simulink model "MyVhclOperator_RTW"  (Simulink 7.5)
settings: Solver=ode1  SolverMode=SingleTasking  StartTime=0.0  StopTime=inf  FixedStep=0.001  RelTol=1e-3
PreLoadFcn:
  | vehicle = 'Car'; if ~length(which('cmcmd')), cmenv; end
  | MyVhclOperator_RTW_bus
InitFcn:
  | vehicle = 'Car'; if ~length(which('cmcmd')), cmenv; end
  | MyVhclOperator_RTW_bus
undefined symbols (not defined in the file or in its folder): OperationFinished, Phase, SteerAng, VCBus
libraries: simulink x45
(part 1 of 3)
Description:
  | CarMaker Real-Time Target (generic)
settings Model: Creator=ml  LastModifiedBy=ml
settings DebuggingCC: SolverPrmCheckMsg=none
settings HardwareCC: TargetHWDeviceType=32-bit Generic  ProdEqTarget=off
settings RTWCC: SystemTargetFile=CarMaker.tlc  TemplateMakefile=CarMaker_unix.tmf  Description=CarMaker Real-Time Target (32-bit)  ProcessScript=CarMaker_make_rtw_hook
settings CodeAppCC: MaxIdLength=127
settings STFCustomTargetCC: ModelReferenceCompliant=off  GeneratePreprocessorConditionals=Disable all  SystemTargetFile=CarMaker.tlc
settings GRTTargetCC: ModelReferenceCompliant=off  ParMdlRefBuildCompliant=off  CompOptLevelCompliant=off  MatFileLogging=off
settings CustomProperty: DataType=string  Value=..
settings EnumStrPairs: String=Car

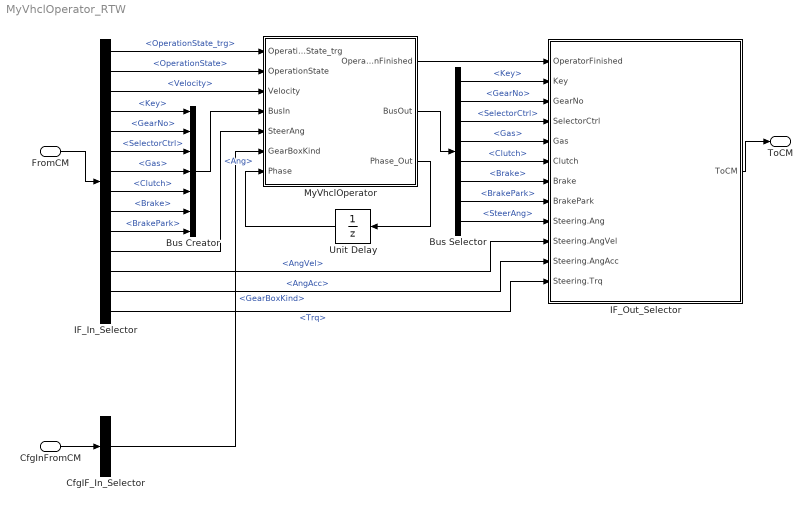
== system MyVhclOperator_RTW ==
  FromCM : Inport  UseBusObject=on
      settings: BusObject=cmVhclOperatorIn
  CfgInFromCM : Inport  Port=2  UseBusObject=on
      settings: BusObject=cmVhclOperatorCfgIn
  Bus Creator : BusCreator  Inputs=7
  Bus Selector : BusSelector  OutputSignals=VCBus.Key,VCBus.GearNo,VCBus.SelectorCtrl,VCBus.Gas,VCBus.Clutch,VCBus.Brake,VCBus.BrakePark,SteerAng
  CfgIF_In_Selector : BusSelector  OutputSignals=GearBoxKind
  IF_In_Selector : BusSelector  OutputSignals=OperationState_trg,OperationState,Velocity,Key,GearNo,SelectorCtrl,Gas,Clutch,Brake,BrakePark,Steering.Ang,Steering.AngVel,Steering.AngAcc,Steering.Trq
  IF_Out_Selector : Subsystem
      settings: OpenFcn=cmSignalSelect('SignalSelection_CB',gcb)
      mask Type: Signal Selection
      mask Description: Signal Selection Block
  MyVhclOperator : Subsystem
  Unit Delay : UnitDelay  SampleTime=-1
  ToCM : Outport  UseBusObject=on
      settings: BusObject=cmVhclOperatorOut
  wires:
  IF_In_Selector/1 -> MyVhclOperator/1(OperationState_trg)  "<OperationState_trg>"
  IF_Out_Selector/1(ToCM) -> ToCM/1
  CfgInFromCM/1 -> CfgIF_In_Selector/1
  CfgIF_In_Selector/1 -> MyVhclOperator/6(GearBoxKind)  "<GearBoxKind>"
  IF_In_Selector/2 -> MyVhclOperator/2(OperationState)  "<OperationState>"
  IF_In_Selector/3 -> MyVhclOperator/3(Velocity)  "<Velocity>"
  MyVhclOperator/3(Phase_Out) -> Unit Delay/1
  Unit Delay/1 -> MyVhclOperator/7(Phase)
  MyVhclOperator/1(OperationFinished) -> IF_Out_Selector/1(OperatorFinished)
  IF_In_Selector/4 -> Bus Creator/1  "<Key>"
  IF_In_Selector/5 -> Bus Creator/2  "<GearNo>"
  IF_In_Selector/6 -> Bus Creator/3  "<SelectorCtrl>"
  IF_In_Selector/7 -> Bus Creator/4  "<Gas>"
  IF_In_Selector/8 -> Bus Creator/5  "<Clutch>"
  IF_In_Selector/9 -> Bus Creator/6  "<Brake>"
  IF_In_Selector/10 -> Bus Creator/7  "<BrakePark>"
  IF_In_Selector/11 -> MyVhclOperator/5(SteerAng)  "<Ang>"
  FromCM/1 -> IF_In_Selector/1
  Bus Creator/1 -> MyVhclOperator/4(BusIn)
  MyVhclOperator/2(BusOut) -> Bus Selector/1
  Bus Selector/1 -> IF_Out_Selector/2(Key)  "<Key>"
  Bus Selector/2 -> IF_Out_Selector/3(GearNo)  "<GearNo>"
  Bus Selector/3 -> IF_Out_Selector/4(SelectorCtrl)  "<SelectorCtrl>"
  Bus Selector/4 -> IF_Out_Selector/5(Gas)  "<Gas>"
  Bus Selector/5 -> IF_Out_Selector/6(Clutch)  "<Clutch>"
  Bus Selector/6 -> IF_Out_Selector/7(Brake)  "<Brake>"
  Bus Selector/7 -> IF_Out_Selector/8(BrakePark)  "<BrakePark>"
  Bus Selector/8 -> IF_Out_Selector/9(Steering.Ang)  "<SteerAng>"
  IF_In_Selector/12 -> IF_Out_Selector/10(Steering.AngVel)  "<AngVel>"
  IF_In_Selector/13 -> IF_Out_Selector/11(Steering.AngAcc)  "<AngAcc>"
  IF_In_Selector/14 -> IF_Out_Selector/12(Steering.Trq)  "<Trq>"

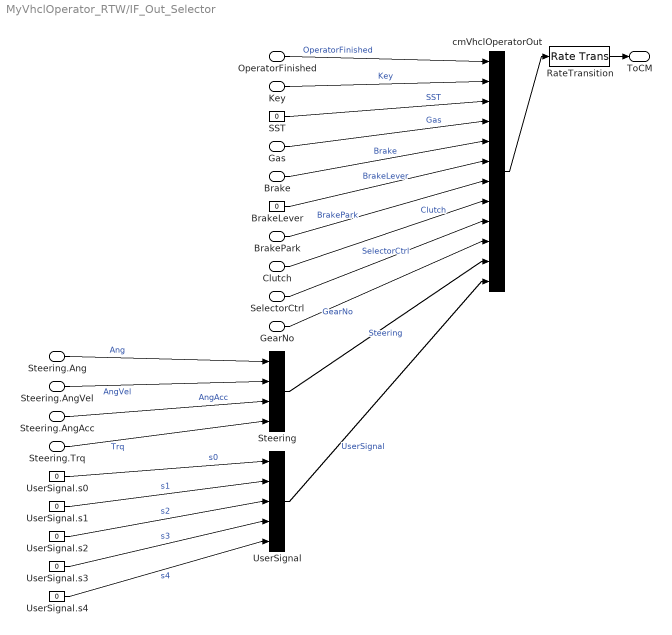
== system MyVhclOperator_RTW/IF_Out_Selector ==
  OperatorFinished : Inport
  Key : Inport  Port=2
  GearNo : Inport  Port=3
  SelectorCtrl : Inport  Port=4
  Gas : Inport  Port=5
  Clutch : Inport  Port=6
  Brake : Inport  Port=7
  BrakePark : Inport  Port=8
  Steering.Ang : Inport  Port=9
  Steering.AngVel : Inport  Port=10
  Steering.AngAcc : Inport  Port=11
  Steering.Trq : Inport  Port=12
  BrakeLever : Constant  Value=0
  RateTransition : RateTransition  OutPortSampleTime=str2num(get_param(bdroot,'FixedStep'))
  SST : Constant  Value=0
  Steering : BusCreator
  UserSignal : BusCreator  Inputs=5
  UserSignal.s{0..4} (5 alike) : Constant  Value=0
  cmVhclOperatorOut : BusCreator  Inputs=12
  ToCM : Outport
  wires:
  RateTransition/1 -> ToCM/1
  cmVhclOperatorOut/1 -> RateTransition/1
  SST/1 -> cmVhclOperatorOut/3  "SST"
  BrakeLever/1 -> cmVhclOperatorOut/6  "BrakeLever"
  Steering/1 -> cmVhclOperatorOut/11  "Steering"
  UserSignal/1 -> cmVhclOperatorOut/12  "UserSignal"
  UserSignal.s0/1 -> UserSignal/1  "s0"
  UserSignal.s1/1 -> UserSignal/2  "s1"
  UserSignal.s2/1 -> UserSignal/3  "s2"
  UserSignal.s3/1 -> UserSignal/4  "s3"
  UserSignal.s4/1 -> UserSignal/5  "s4"
  OperatorFinished/1 -> cmVhclOperatorOut/1  "OperatorFinished"
  Key/1 -> cmVhclOperatorOut/2  "Key"
  GearNo/1 -> cmVhclOperatorOut/10  "GearNo"
  SelectorCtrl/1 -> cmVhclOperatorOut/9  "SelectorCtrl"
  Gas/1 -> cmVhclOperatorOut/4  "Gas"
  Clutch/1 -> cmVhclOperatorOut/8  "Clutch"
  Brake/1 -> cmVhclOperatorOut/5  "Brake"
  BrakePark/1 -> cmVhclOperatorOut/7  "BrakePark"
  Steering.Ang/1 -> Steering/1  "Ang"
  Steering.AngVel/1 -> Steering/2  "AngVel"
  Steering.AngAcc/1 -> Steering/3  "AngAcc"
  Steering.Trq/1 -> Steering/4  "Trq"

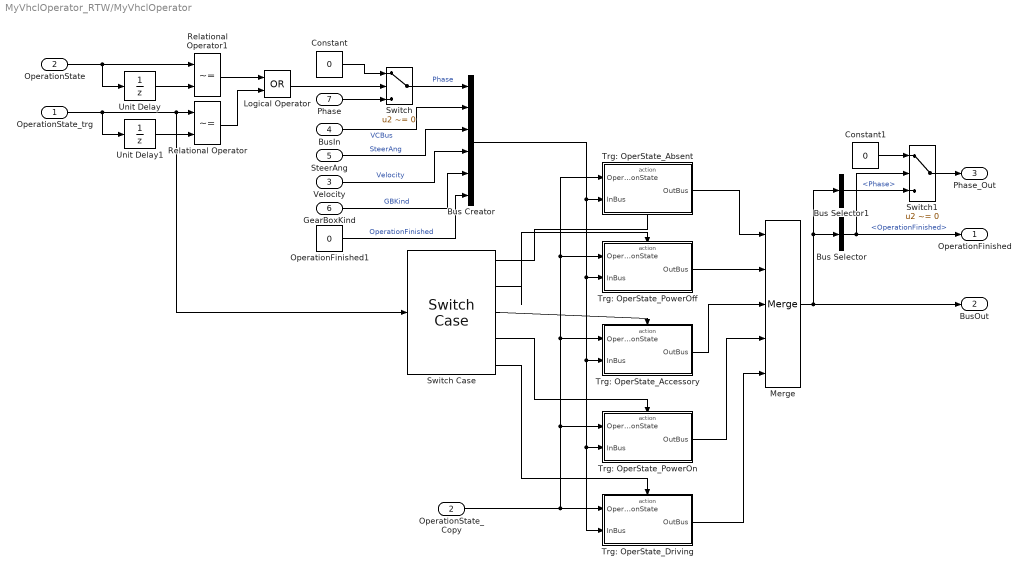
== system MyVhclOperator_RTW/MyVhclOperator ==
  OperationState_trg : Inport  OutDataType=fixdt(1, 16)  OutScaling=2^0
  OperationState : Inport  Port=2  OutDataType=fixdt(1, 16)  OutScaling=2^0
  Velocity : Inport  Port=3  OutDataType=fixdt(1, 16)  OutScaling=2^0
  BusIn : Inport  Port=4  OutDataType=fixdt(1, 16)  OutScaling=2^0
  SteerAng : Inport  Port=5  OutDataType=fixdt(1, 16)  OutScaling=2^0
  GearBoxKind : Inport  Port=6  OutDataType=fixdt(1, 16)  OutScaling=2^0
  Phase : Inport  Port=7  OutDataType=fixdt(1, 16)  OutScaling=2^0
  Bus Creator : BusCreator  Inputs=6
  Bus Selector : BusSelector  OutputSignals=OperationFinished
  Bus Selector1 : BusSelector  OutputSignals=Phase
  Constant : Constant  Value=0  OutDataType=fixdt(1, 16)  OutScaling=2^0
  Constant1 : Constant  Value=0  OutDataType=fixdt(1, 16)  OutScaling=2^0
  Logical Operator : Logic  Operator=OR  AllPortsSameDT=off  OutDataTypeMode=boolean  LogicDataType=fixdt(0, 8)  OutDataTypeStr=boolean
  Merge : Merge  Inputs=5
  OperationFinished1 : Constant  Value=0  OutDataType=fixdt(1, 16)  OutScaling=2^0
  OperationState_Copy : InportShadow  Port=2  OutDataType=fixdt(1, 16)  OutScaling=2^0
  Relational Operator : RelationalOperator  Operator=~=  LogicOutDataTypeMode=boolean  LogicDataType=fixdt(0, 8)  OutDataTypeStr=boolean
  Relational Operator1 : RelationalOperator  Operator=~=  LogicOutDataTypeMode=boolean  LogicDataType=fixdt(0, 8)  OutDataTypeStr=boolean
  Switch : Switch  Criteria=u2 ~= 0  OutDataType=fixdt(1, 16)  OutScaling=2^0
  Switch Case : SwitchCase  CaseConditions={0,1,2,3,4}  ShowDefaultCase=off
  Switch1 : Switch  Criteria=u2 ~= 0  OutDataType=fixdt(1, 16)  OutScaling=2^0
  Trg: OperState_Absent : Subsystem  TreatAsAtomicUnit=on
  Trg: OperState_Accessory : Subsystem  TreatAsAtomicUnit=on
  Trg: OperState_Driving : Subsystem  TreatAsAtomicUnit=on
  Trg: OperState_PowerOff : Subsystem  TreatAsAtomicUnit=on
  Trg: OperState_PowerOn : Subsystem  TreatAsAtomicUnit=on
  Unit Delay : UnitDelay  SampleTime=-1
  Unit Delay1 : UnitDelay  SampleTime=-1
  OperationFinished : Outport  OutDataType=fixdt(1, 16)  OutScaling=2^0
  BusOut : Outport  Port=2  OutDataType=fixdt(1, 16)  OutScaling=2^0
  Phase_Out : Outport  Port=3  OutDataType=fixdt(1, 16)  OutScaling=2^0
  wires:
  Switch/1 -> Bus Creator/1  "Phase"
  OperationState_trg/1 -> Relational Operator/1, Switch Case/1, Unit Delay1/1
  OperationState/1 -> Relational Operator1/1, Unit Delay/1
  Logical Operator/1 -> Switch/2
  Constant/1 -> Switch/1
  Switch Case/1 -> Trg: OperState_Absent/Action
  Switch Case/2 -> Trg: OperState_PowerOff/Action
  Switch Case/3 -> Trg: OperState_Accessory/Action
  Switch Case/4 -> Trg: OperState_PowerOn/Action
  Switch Case/5 -> Trg: OperState_Driving/Action
  Trg: OperState_Absent/1(OutBus) -> Merge/1
  Trg: OperState_PowerOff/1(OutBus) -> Merge/2
  Trg: OperState_Accessory/1(OutBus) -> Merge/3
  Trg: OperState_PowerOn/1(OutBus) -> Merge/4
  Trg: OperState_Driving/1(OutBus) -> Merge/5
  OperationState_Copy/1 -> Trg: OperState_PowerOff/1(OperationState), Trg: OperState_Absent/1(OperationState), Trg: OperState_Accessory/1(OperationState), Trg: OperState_PowerOn/1(OperationState), Trg: OperState_Driving/1(OperationState)
  Bus Creator/1 -> Trg: OperState_Absent/2(InBus), Trg: OperState_PowerOn/2(InBus), Trg: OperState_Driving/2(InBus), Trg: OperState_Accessory/2(InBus), Trg: OperState_PowerOff/2(InBus)
  Relational Operator1/1 -> Logical Operator/1
  Relational Operator/1 -> Logical Operator/2
  Unit Delay/1 -> Relational Operator1/2
  Unit Delay1/1 -> Relational Operator/2
  Phase/1 -> Switch/3
  BusIn/1 -> Bus Creator/2  "VCBus"
  SteerAng/1 -> Bus Creator/3  "SteerAng"
  Velocity/1 -> Bus Creator/4  "Velocity"
  GearBoxKind/1 -> Bus Creator/5  "GBKind"
  OperationFinished1/1 -> Bus Creator/6  "OperationFinished"
  Bus Selector/1 -> OperationFinished/1, Switch1/2  "<OperationFinished>"
  Switch1/1 -> Phase_Out/1
  Bus Selector1/1 -> Switch1/3  "<Phase>"
  Constant1/1 -> Switch1/1
  Merge/1 -> Bus Selector/1, Bus Selector1/1, BusOut/1

== system MyVhclOperator_RTW/MyVhclOperator/Trg: OperState_Absent ==
  note: Trg: OperState_Absent
  OperationState : Inport  OutDataType=fixdt(1, 16)  OutScaling=2^0
  InBus : Inport  Port=2  OutDataType=fixdt(1, 16)  OutScaling=2^0
  Action Port : ActionPort  ActionType=case
  Merge : Merge  Inputs=5
  OperState_Absent : Subsystem  TreatAsAtomicUnit=on
  OperState_Driving : Subsystem  TreatAsAtomicUnit=on
  OperState_PowerAccessory : Subsystem  TreatAsAtomicUnit=on
  OperState_PowerOff : Subsystem  TreatAsAtomicUnit=on
  OperState_PowerOn : Subsystem  TreatAsAtomicUnit=on
  Switch Case : SwitchCase  CaseConditions={0,1,2,3,4}  ShowDefaultCase=off
  OutBus : Outport  OutDataType=fixdt(1, 16)  OutScaling=2^0  InitialOutput=[0]
  wires:
  OperationState/1 -> Switch Case/1
  Switch Case/1 -> OperState_Absent/Action
  Switch Case/2 -> OperState_PowerOff/Action
  Switch Case/3 -> OperState_PowerAccessory/Action
  Switch Case/4 -> OperState_PowerOn/Action
  Switch Case/5 -> OperState_Driving/Action
  InBus/1 -> OperState_Absent/1(InBus), OperState_PowerOff/1(InBus), OperState_PowerAccessory/1(InBus), OperState_PowerOn/1(InBus), OperState_Driving/1(InBus)
  OperState_Absent/1(OutBus) -> Merge/1
  OperState_PowerOff/1(OutBus) -> Merge/2
  OperState_PowerAccessory/1(OutBus) -> Merge/3
  OperState_PowerOn/1(OutBus) -> Merge/4
  OperState_Driving/1(OutBus) -> Merge/5
  Merge/1 -> OutBus/1

== system MyVhclOperator_RTW/MyVhclOperator/Trg: OperState_Accessory ==
  note: Trg: OperState_Accessory
  OperationState : Inport  OutDataType=fixdt(1, 16)  OutScaling=2^0
  InBus : Inport  Port=2  OutDataType=fixdt(1, 16)  OutScaling=2^0
  Action Port : ActionPort  ActionType=case
  Merge : Merge  Inputs=5
  OperState_Absent : Subsystem  TreatAsAtomicUnit=on
  OperState_Accessory : Subsystem  TreatAsAtomicUnit=on
  OperState_Driving : Subsystem  TreatAsAtomicUnit=on
  OperState_PowerOff : Subsystem  TreatAsAtomicUnit=on
  OperState_PowerOn : Subsystem  TreatAsAtomicUnit=on
  Switch Case : SwitchCase  CaseConditions={0,1,2,3,4}  ShowDefaultCase=off
  OutBus : Outport  OutDataType=fixdt(1, 16)  OutScaling=2^0  InitialOutput=[0]
  wires:
  Merge/1 -> OutBus/1
  OperState_Driving/1(OutBus) -> Merge/5
  OperState_PowerOn/1(OutBus) -> Merge/4
  OperState_Accessory/1(OutBus) -> Merge/3
  OperState_PowerOff/1(OutBus) -> Merge/2
  OperState_Absent/1(OutBus) -> Merge/1
  InBus/1 -> OperState_PowerOff/1(InBus), OperState_Absent/1(InBus), OperState_Accessory/1(InBus), OperState_PowerOn/1(InBus), OperState_Driving/1(InBus)
  Switch Case/5 -> OperState_Driving/Action
  Switch Case/4 -> OperState_PowerOn/Action
  Switch Case/3 -> OperState_Accessory/Action
  Switch Case/2 -> OperState_PowerOff/Action
  Switch Case/1 -> OperState_Absent/Action
  OperationState/1 -> Switch Case/1

== system MyVhclOperator_RTW/MyVhclOperator/Trg: OperState_Driving ==
  note: Trg: OperState_Driving
  OperationState : Inport  OutDataType=fixdt(1, 16)  OutScaling=2^0
  InBus : Inport  Port=2  OutDataType=fixdt(1, 16)  OutScaling=2^0
  Action Port : ActionPort  ActionType=case
  Merge : Merge  Inputs=5
  OperState_Absent : Subsystem  TreatAsAtomicUnit=on
  OperState_Driving : Subsystem  TreatAsAtomicUnit=on
  OperState_PowerAccessory : Subsystem  TreatAsAtomicUnit=on
  OperState_PowerOff : Subsystem  TreatAsAtomicUnit=on
  OperState_PowerOn : Subsystem  TreatAsAtomicUnit=on
  Switch Case : SwitchCase  CaseConditions={0,1,2,3,4}  ShowDefaultCase=off
  OutBus : Outport  OutDataType=fixdt(1, 16)  OutScaling=2^0  InitialOutput=[0]
  wires:
  Merge/1 -> OutBus/1
  OperState_Driving/1(OutBus) -> Merge/5
  OperState_PowerOn/1(OutBus) -> Merge/4
  OperState_PowerAccessory/1(OutBus) -> Merge/3
  OperState_PowerOff/1(OutBus) -> Merge/2
  OperState_Absent/1(OutBus) -> Merge/1
  InBus/1 -> OperState_Absent/1(InBus), OperState_PowerOff/1(InBus), OperState_PowerAccessory/1(InBus), OperState_PowerOn/1(InBus), OperState_Driving/1(InBus)
  Switch Case/5 -> OperState_Driving/Action
  Switch Case/4 -> OperState_PowerOn/Action
  Switch Case/3 -> OperState_PowerAccessory/Action
  Switch Case/2 -> OperState_PowerOff/Action
  Switch Case/1 -> OperState_Absent/Action
  OperationState/1 -> Switch Case/1

== system MyVhclOperator_RTW/MyVhclOperator/Trg: OperState_PowerOff ==
  note: Trg: OperState_PowerOff
  OperationState : Inport  OutDataType=fixdt(1, 16)  OutScaling=2^0
  InBus : Inport  Port=2  OutDataType=fixdt(1, 16)  OutScaling=2^0
  Action Port : ActionPort  ActionType=case
  Merge : Merge  Inputs=5
  OperState_Absent : Subsystem  TreatAsAtomicUnit=on
  OperState_Driving : Subsystem  TreatAsAtomicUnit=on
  OperState_PowerAccessory : Subsystem  TreatAsAtomicUnit=on
  OperState_PowerOff : Subsystem  TreatAsAtomicUnit=on
  OperState_PowerOn : Subsystem  TreatAsAtomicUnit=on
  Switch Case : SwitchCase  CaseConditions={0,1,2,3,4}  ShowDefaultCase=off
  OutBus : Outport  OutDataType=fixdt(1, 16)  OutScaling=2^0  InitialOutput=[0]
  wires:
  OperationState/1 -> Switch Case/1
  Switch Case/1 -> OperState_Absent/Action
  Switch Case/2 -> OperState_PowerOff/Action
  Switch Case/3 -> OperState_PowerAccessory/Action
  Switch Case/4 -> OperState_PowerOn/Action
  Switch Case/5 -> OperState_Driving/Action
  InBus/1 -> OperState_PowerOff/1(InBus), OperState_Absent/1(InBus), OperState_PowerAccessory/1(InBus), OperState_PowerOn/1(InBus), OperState_Driving/1(InBus)
  OperState_Absent/1(OutBus) -> Merge/1
  OperState_PowerOff/1(OutBus) -> Merge/2
  OperState_PowerAccessory/1(OutBus) -> Merge/3
  OperState_PowerOn/1(OutBus) -> Merge/4
  OperState_Driving/1(OutBus) -> Merge/5
  Merge/1 -> OutBus/1

== system MyVhclOperator_RTW/MyVhclOperator/Trg: OperState_PowerOn ==
  note: Trg: OperState_PowerOn
  OperationState : Inport  OutDataType=fixdt(1, 16)  OutScaling=2^0
  InBus : Inport  Port=2  OutDataType=fixdt(1, 16)  OutScaling=2^0
  Action Port : ActionPort  ActionType=case
  Merge : Merge  Inputs=5
  OperState_Absent : Subsystem  TreatAsAtomicUnit=on
  OperState_Driving : Subsystem  TreatAsAtomicUnit=on
  OperState_PowerAccessory : Subsystem  TreatAsAtomicUnit=on
  OperState_PowerOff : Subsystem  TreatAsAtomicUnit=on
  OperState_PowerOn : Subsystem  TreatAsAtomicUnit=on
  Switch Case : SwitchCase  CaseConditions={0,1,2,3,4}  ShowDefaultCase=off
  OutBus : Outport  OutDataType=fixdt(1, 16)  OutScaling=2^0  InitialOutput=[0]
  wires:
  OperationState/1 -> Switch Case/1
  Switch Case/1 -> OperState_Absent/Action
  Switch Case/2 -> OperState_PowerOff/Action
  Switch Case/3 -> OperState_PowerAccessory/Action
  Switch Case/4 -> OperState_PowerOn/Action
  Switch Case/5 -> OperState_Driving/Action
  InBus/1 -> OperState_PowerOn/1(InBus), OperState_PowerAccessory/1(InBus), OperState_Absent/1(InBus), OperState_PowerOff/1(InBus), OperState_Driving/1(InBus)
  OperState_Absent/1(OutBus) -> Merge/1
  OperState_PowerOff/1(OutBus) -> Merge/2
  OperState_PowerAccessory/1(OutBus) -> Merge/3
  OperState_PowerOn/1(OutBus) -> Merge/4
  OperState_Driving/1(OutBus) -> Merge/5
  Merge/1 -> OutBus/1

== system MyVhclOperator_RTW/MyVhclOperator/Trg: OperState_Absent/OperState_Absent ==
  InBus : Inport  OutDataType=fixdt(1, 16)  OutScaling=2^0
  Action Port : ActionPort  ActionType=case
  Bus Assignment : BusAssignment  AssignedSignals=VCBus.Key,VCBus.GearNo,VCBus.SelectorCtrl,VCBus.Gas,VCBus.Clutch,VCBus.Brake,VCBus.BrakePark,Phase,OperationFinished
  Bus Selector : BusSelector  OutputSignals=GBKind
  Bus Selector1 : BusSelector  OutputSignals=Key,GearNo,SelectorCtrl,Gas,Clutch,Brake,BrakePark
  OperState: Absent : Subsystem
  OperationFinished : Constant  OutDataType=fixdt(1, 16)  OutScaling=2^0
  Phase : Constant  Value=0  OutDataType=fixdt(1, 16)  OutScaling=2^0
  Signal Conversion : SignalConversion  ConversionOutput=Bus copy
  OutBus : Outport  OutDataType=fixdt(1, 16)  OutScaling=2^0  InitialOutput=[0]
  wires:
  InBus/1 -> Bus Selector/1, Signal Conversion/1
  Bus Selector/1 -> OperState: Absent/1(GBKind)  "<GBKind>"
  Bus Assignment/1 -> OutBus/1
  OperationFinished/1 -> Bus Assignment/10
  Phase/1 -> Bus Assignment/9
  OperState: Absent/1(BusOut) -> Bus Selector1/1  "VC_Bus"
  Signal Conversion/1 -> Bus Assignment/1
  Bus Selector1/1 -> Bus Assignment/2  "<Key>"
  Bus Selector1/2 -> Bus Assignment/3  "<GearNo>"
  Bus Selector1/3 -> Bus Assignment/4  "<SelectorCtrl>"
  Bus Selector1/4 -> Bus Assignment/5  "<Gas>"
  Bus Selector1/5 -> Bus Assignment/6  "<Clutch>"
  Bus Selector1/6 -> Bus Assignment/7  "<Brake>"
  Bus Selector1/7 -> Bus Assignment/8  "<BrakePark>"

== system MyVhclOperator_RTW/MyVhclOperator/Trg: OperState_Absent/OperState_Driving ==
  InBus : Inport  OutDataType=fixdt(1, 16)  OutScaling=2^0
  Action Port : ActionPort  ActionType=case
  Drive2Off : Subsystem
  OutBus : Outport  OutDataType=fixdt(1, 16)  OutScaling=2^0
  wires:
  Drive2Off/1(BusOut) -> OutBus/1
  InBus/1 -> Drive2Off/1(BusIn)

== system MyVhclOperator_RTW/MyVhclOperator/Trg: OperState_Absent/OperState_PowerAccessory ==
  InBus : Inport  OutDataType=fixdt(1, 16)  OutScaling=2^0
  Action Port : ActionPort  ActionType=case
  Bus Assignment1 : BusAssignment  AssignedSignals=VCBus.Key,VCBus.GearNo,VCBus.SelectorCtrl,VCBus.Gas,VCBus.Clutch,VCBus.Brake,VCBus.BrakePark,Phase
  Bus Selector : BusSelector  OutputSignals=GBKind,Phase
  Bus Selector1 : BusSelector  OutputSignals=Key,GearNo,SelectorCtrl,Gas,Clutch,Brake,BrakePark
  OperState: PowerOn : Subsystem
  SetOutputAndWait : Subsystem
  Signal Conversion : SignalConversion  ConversionOutput=Bus copy
  OutBus : Outport  OutDataType=fixdt(1, 16)  OutScaling=2^0  InitialOutput=[0]
  wires:
  InBus/1 -> Bus Selector/1, Signal Conversion/1
  Bus Selector/1 -> OperState: PowerOn/1(GBKind)  "<GBKind>"
  Bus Assignment1/1 -> OutBus/1
  Bus Selector/2 -> SetOutputAndWait/1(PhaseIn)  "<Phase>"
  OperState: PowerOn/1(BusOut) -> Bus Selector1/1  "VC_Bus"
  SetOutputAndWait/1(PhaseOut) -> Bus Assignment1/9
  Signal Conversion/1 -> Bus Assignment1/1
  Bus Selector1/1 -> Bus Assignment1/2  "<Key>"
  Bus Selector1/2 -> Bus Assignment1/3  "<GearNo>"
  Bus Selector1/3 -> Bus Assignment1/4  "<SelectorCtrl>"
  Bus Selector1/4 -> Bus Assignment1/5  "<Gas>"
  Bus Selector1/5 -> Bus Assignment1/6  "<Clutch>"
  Bus Selector1/6 -> Bus Assignment1/7  "<Brake>"
  Bus Selector1/7 -> Bus Assignment1/8  "<BrakePark>"

== system MyVhclOperator_RTW/MyVhclOperator/Trg: OperState_Absent/OperState_PowerOff ==
  InBus : Inport  OutDataType=fixdt(1, 16)  OutScaling=2^0
  Action Port : ActionPort  ActionType=case
  Bus Assignment1 : BusAssignment  AssignedSignals=VCBus.Key,VCBus.GearNo,VCBus.SelectorCtrl,VCBus.Gas,VCBus.Clutch,VCBus.Brake,VCBus.BrakePark,Phase
  Bus Selector : BusSelector  OutputSignals=GBKind,Phase
  Bus Selector1 : BusSelector  OutputSignals=Key,GearNo,SelectorCtrl,Gas,Clutch,Brake,BrakePark
  OperState: Absent : Subsystem
  SetOutputAndWait : Subsystem
  Signal Conversion : SignalConversion  ConversionOutput=Bus copy
  OutBus : Outport  OutDataType=fixdt(1, 16)  OutScaling=2^0  InitialOutput=[0]
  wires:
  InBus/1 -> Bus Selector/1, Signal Conversion/1
  Bus Selector/1 -> OperState: Absent/1(GBKind)  "<GBKind>"
  Bus Assignment1/1 -> OutBus/1
  OperState: Absent/1(BusOut) -> Bus Selector1/1  "VC_Bus"
  Bus Selector/2 -> SetOutputAndWait/1(PhaseIn)  "<Phase>"
  SetOutputAndWait/1(PhaseOut) -> Bus Assignment1/9
  Signal Conversion/1 -> Bus Assignment1/1
  Bus Selector1/1 -> Bus Assignment1/2  "<Key>"
  Bus Selector1/2 -> Bus Assignment1/3  "<GearNo>"
  Bus Selector1/3 -> Bus Assignment1/4  "<SelectorCtrl>"
  Bus Selector1/4 -> Bus Assignment1/5  "<Gas>"
  Bus Selector1/5 -> Bus Assignment1/6  "<Clutch>"
  Bus Selector1/6 -> Bus Assignment1/7  "<Brake>"
  Bus Selector1/7 -> Bus Assignment1/8  "<BrakePark>"

== system MyVhclOperator_RTW/MyVhclOperator/Trg: OperState_Absent/OperState_PowerOn ==
  InBus : Inport  OutDataType=fixdt(1, 16)  OutScaling=2^0
  Action Port : ActionPort  ActionType=case
  Bus Assignment1 : BusAssignment  AssignedSignals=VCBus.Key,VCBus.GearNo,VCBus.SelectorCtrl,VCBus.Gas,VCBus.Clutch,VCBus.Brake,VCBus.BrakePark,Phase
  Bus Selector : BusSelector  OutputSignals=GBKind,Phase
  Bus Selector1 : BusSelector  OutputSignals=Key,GearNo,SelectorCtrl,Gas,Clutch,Brake,BrakePark
  OperState: PowerOff : Subsystem
  SetOutputAndWait : Subsystem
  Signal Conversion : SignalConversion  ConversionOutput=Bus copy
  OutBus : Outport  OutDataType=fixdt(1, 16)  OutScaling=2^0  InitialOutput=[0]
  wires:
  Bus Selector/2 -> SetOutputAndWait/1(PhaseIn)  "<Phase>"
  Bus Selector/1 -> OperState: PowerOff/1(GBKind)  "<GBKind>"
  InBus/1 -> Bus Selector/1, Signal Conversion/1
  OperState: PowerOff/1(BusOut) -> Bus Selector1/1  "VC_Bus"
  SetOutputAndWait/1(PhaseOut) -> Bus Assignment1/9
  Bus Assignment1/1 -> OutBus/1
  Signal Conversion/1 -> Bus Assignment1/1
  Bus Selector1/1 -> Bus Assignment1/2  "<Key>"
  Bus Selector1/2 -> Bus Assignment1/3  "<GearNo>"
  Bus Selector1/3 -> Bus Assignment1/4  "<SelectorCtrl>"
  Bus Selector1/4 -> Bus Assignment1/5  "<Gas>"
  Bus Selector1/5 -> Bus Assignment1/6  "<Clutch>"
  Bus Selector1/6 -> Bus Assignment1/7  "<Brake>"
  Bus Selector1/7 -> Bus Assignment1/8  "<BrakePark>"

== system MyVhclOperator_RTW/MyVhclOperator/Trg: OperState_Accessory/OperState_Absent ==
  InBus : Inport  OutDataType=fixdt(1, 16)  OutScaling=2^0
  Action Port : ActionPort  ActionType=case
  Bus Assignment : BusAssignment  AssignedSignals=VCBus.Key,VCBus.GearNo,VCBus.SelectorCtrl,VCBus.Gas,VCBus.Clutch,VCBus.Brake,VCBus.BrakePark
  Bus Selector : BusSelector  OutputSignals=GBKind
  Bus Selector1 : BusSelector  OutputSignals=Key,GearNo,SelectorCtrl,Gas,Clutch,Brake,BrakePark
  OperState: PowerOff : Subsystem
  Signal Conversion : SignalConversion  ConversionOutput=Bus copy
  OutBus : Outport  OutDataType=fixdt(1, 16)  OutScaling=2^0  InitialOutput=[0]
  wires:
  OperState: PowerOff/1(BusOut) -> Bus Selector1/1  "VC_Bus"
  Bus Assignment/1 -> OutBus/1
  Bus Selector/1 -> OperState: PowerOff/1(GBKind)  "<GBKind>"
  InBus/1 -> Bus Selector/1, Signal Conversion/1
  Signal Conversion/1 -> Bus Assignment/1
  Bus Selector1/1 -> Bus Assignment/2  "<Key>"
  Bus Selector1/2 -> Bus Assignment/3  "<GearNo>"
  Bus Selector1/3 -> Bus Assignment/4  "<SelectorCtrl>"
  Bus Selector1/4 -> Bus Assignment/5  "<Gas>"
  Bus Selector1/5 -> Bus Assignment/6  "<Clutch>"
  Bus Selector1/6 -> Bus Assignment/7  "<Brake>"
  Bus Selector1/7 -> Bus Assignment/8  "<BrakePark>"

== system MyVhclOperator_RTW/MyVhclOperator/Trg: OperState_Accessory/OperState_Accessory ==
  InBus : Inport  OutDataType=fixdt(1, 16)  OutScaling=2^0
  Action Port : ActionPort  ActionType=case
  Bus Assignment1 : BusAssignment  AssignedSignals=VCBus.Key,VCBus.GearNo,VCBus.SelectorCtrl,VCBus.Gas,VCBus.Clutch,VCBus.Brake,VCBus.BrakePark,Phase,OperationFinished
  Bus Selector : BusSelector  OutputSignals=GBKind
  Bus Selector1 : BusSelector  OutputSignals=Key,GearNo,SelectorCtrl,Gas,Clutch,Brake,BrakePark
  OperState: PowerAcc : Subsystem
  OperationFinished : Constant  OutDataType=fixdt(1, 16)  OutScaling=2^0
  Phase : Constant  Value=0  OutDataType=fixdt(1, 16)  OutScaling=2^0
  Signal Conversion : SignalConversion  ConversionOutput=Bus copy
  OutBus : Outport  OutDataType=fixdt(1, 16)  OutScaling=2^0  InitialOutput=[0]
  wires:
  Bus Assignment1/1 -> OutBus/1
  Bus Selector/1 -> OperState: PowerAcc/1(GBKind)  "<GBKind>"
  InBus/1 -> Bus Selector/1, Signal Conversion/1
  OperationFinished/1 -> Bus Assignment1/10
  Phase/1 -> Bus Assignment1/9
  OperState: PowerAcc/1(BusOut) -> Bus Selector1/1  "VC_Bus"
  Signal Conversion/1 -> Bus Assignment1/1
  Bus Selector1/1 -> Bus Assignment1/2  "<Key>"
  Bus Selector1/2 -> Bus Assignment1/3  "<GearNo>"
  Bus Selector1/3 -> Bus Assignment1/4  "<SelectorCtrl>"
  Bus Selector1/4 -> Bus Assignment1/5  "<Gas>"
  Bus Selector1/5 -> Bus Assignment1/6  "<Clutch>"
  Bus Selector1/6 -> Bus Assignment1/7  "<Brake>"
  Bus Selector1/7 -> Bus Assignment1/8  "<BrakePark>"

== system MyVhclOperator_RTW/MyVhclOperator/Trg: OperState_Accessory/OperState_Driving ==
  InBus : Inport  OutDataType=fixdt(1, 16)  OutScaling=2^0
  Action Port : ActionPort  ActionType=case
  Drive2Off : Subsystem
  OutBus : Outport  OutDataType=fixdt(1, 16)  OutScaling=2^0
  wires:
  Drive2Off/1(BusOut) -> OutBus/1
  InBus/1 -> Drive2Off/1(BusIn)

== system MyVhclOperator_RTW/MyVhclOperator/Trg: OperState_Accessory/OperState_PowerOff ==
  InBus : Inport  OutDataType=fixdt(1, 16)  OutScaling=2^0
  Action Port : ActionPort  ActionType=case
  Bus Assignment1 : BusAssignment  AssignedSignals=VCBus.Key,VCBus.GearNo,VCBus.SelectorCtrl,VCBus.Gas,VCBus.Clutch,VCBus.Brake,VCBus.BrakePark,Phase
  Bus Selector : BusSelector  OutputSignals=GBKind,Phase
  Bus Selector1 : BusSelector  OutputSignals=Key,GearNo,SelectorCtrl,Gas,Clutch,Brake,BrakePark
  OperState: PowerAcc : Subsystem
  SetOutputAndWait : Subsystem
  Signal Conversion : SignalConversion  ConversionOutput=Bus copy
  OutBus : Outport  OutDataType=fixdt(1, 16)  OutScaling=2^0  InitialOutput=[0]
  wires:
  Bus Selector/2 -> SetOutputAndWait/1(PhaseIn)  "<Phase>"
  Bus Assignment1/1 -> OutBus/1
  Bus Selector/1 -> OperState: PowerAcc/1(GBKind)  "<GBKind>"
  InBus/1 -> Bus Selector/1, Signal Conversion/1
  SetOutputAndWait/1(PhaseOut) -> Bus Assignment1/9
  OperState: PowerAcc/1(BusOut) -> Bus Selector1/1  "VC_Bus"
  Signal Conversion/1 -> Bus Assignment1/1
  Bus Selector1/1 -> Bus Assignment1/2  "<Key>"
  Bus Selector1/2 -> Bus Assignment1/3  "<GearNo>"
  Bus Selector1/3 -> Bus Assignment1/4  "<SelectorCtrl>"
  Bus Selector1/4 -> Bus Assignment1/5  "<Gas>"
  Bus Selector1/5 -> Bus Assignment1/6  "<Clutch>"
  Bus Selector1/6 -> Bus Assignment1/7  "<Brake>"
  Bus Selector1/7 -> Bus Assignment1/8  "<BrakePark>"

== system MyVhclOperator_RTW/MyVhclOperator/Trg: OperState_Accessory/OperState_PowerOn ==
  InBus : Inport  OutDataType=fixdt(1, 16)  OutScaling=2^0
  Action Port : ActionPort  ActionType=case
  Bus Assignment1 : BusAssignment  AssignedSignals=VCBus.Key,VCBus.GearNo,VCBus.SelectorCtrl,VCBus.Gas,VCBus.Clutch,VCBus.Brake,VCBus.BrakePark,Phase
  Bus Selector : BusSelector  OutputSignals=GBKind,Phase
  Bus Selector1 : BusSelector  OutputSignals=Key,GearNo,SelectorCtrl,Gas,Clutch,Brake,BrakePark
  OperState: PowerOff : Subsystem
  SetOutputAndWait : Subsystem
  Signal Conversion : SignalConversion  ConversionOutput=Bus copy
  OutBus : Outport  OutDataType=fixdt(1, 16)  OutScaling=2^0  InitialOutput=[0]
  wires:
  Bus Selector/2 -> SetOutputAndWait/1(PhaseIn)  "<Phase>"
  Bus Selector/1 -> OperState: PowerOff/1(GBKind)  "<GBKind>"
  InBus/1 -> Bus Selector/1, Signal Conversion/1
  OperState: PowerOff/1(BusOut) -> Bus Selector1/1  "VC_Bus"
  SetOutputAndWait/1(PhaseOut) -> Bus Assignment1/9
  Bus Assignment1/1 -> OutBus/1
  Signal Conversion/1 -> Bus Assignment1/1
  Bus Selector1/1 -> Bus Assignment1/2  "<Key>"
  Bus Selector1/2 -> Bus Assignment1/3  "<GearNo>"
  Bus Selector1/3 -> Bus Assignment1/4  "<SelectorCtrl>"
  Bus Selector1/4 -> Bus Assignment1/5  "<Gas>"
  Bus Selector1/5 -> Bus Assignment1/6  "<Clutch>"
  Bus Selector1/6 -> Bus Assignment1/7  "<Brake>"
  Bus Selector1/7 -> Bus Assignment1/8  "<BrakePark>"

== system MyVhclOperator_RTW/MyVhclOperator/Trg: OperState_Driving/OperState_Absent ==
  InBus : Inport  OutDataType=fixdt(1, 16)  OutScaling=2^0
  Action Port : ActionPort  ActionType=case
  Bus Assignment : BusAssignment  AssignedSignals=VCBus.Key,VCBus.GearNo,VCBus.SelectorCtrl,VCBus.Gas,VCBus.Clutch,VCBus.Brake,VCBus.BrakePark
  Bus Selector : BusSelector  OutputSignals=GBKind
  Bus Selector1 : BusSelector  OutputSignals=Key,GearNo,SelectorCtrl,Gas,Clutch,Brake,BrakePark
  OperState: PowerOff : Subsystem
  Signal Conversion : SignalConversion  ConversionOutput=Bus copy
  OutBus : Outport  OutDataType=fixdt(1, 16)  OutScaling=2^0  InitialOutput=[0]
  wires:
  InBus/1 -> Bus Selector/1, Signal Conversion/1
  Bus Selector/1 -> OperState: PowerOff/1(GBKind)  "<GBKind>"
  Bus Assignment/1 -> OutBus/1
  OperState: PowerOff/1(BusOut) -> Bus Selector1/1  "VC_Bus"
  Signal Conversion/1 -> Bus Assignment/1
  Bus Selector1/1 -> Bus Assignment/2  "<Key>"
  Bus Selector1/2 -> Bus Assignment/3  "<GearNo>"
  Bus Selector1/3 -> Bus Assignment/4  "<SelectorCtrl>"
  Bus Selector1/4 -> Bus Assignment/5  "<Gas>"
  Bus Selector1/5 -> Bus Assignment/6  "<Clutch>"
  Bus Selector1/6 -> Bus Assignment/7  "<Brake>"
  Bus Selector1/7 -> Bus Assignment/8  "<BrakePark>"

== system MyVhclOperator_RTW/MyVhclOperator/Trg: OperState_Driving/OperState_Driving ==
  InBus : Inport  OutDataType=fixdt(1, 16)  OutScaling=2^0
  Action Port : ActionPort  ActionType=case
  Bus Assignment1 : BusAssignment  AssignedSignals=VCBus.Key,VCBus.GearNo,VCBus.SelectorCtrl,VCBus.Gas,VCBus.Clutch,VCBus.Brake,VCBus.BrakePark,Phase,OperationFinished
  Bus Selector : BusSelector  OutputSignals=GBKind
  Bus Selector1 : BusSelector  OutputSignals=Key,GearNo,SelectorCtrl,Gas,Clutch,Brake,BrakePark
  OperState: Driving : Subsystem
  OperationFinished : Constant  OutDataType=fixdt(1, 16)  OutScaling=2^0
  Phase : Constant  Value=0  OutDataType=fixdt(1, 16)  OutScaling=2^0
  Signal Conversion : SignalConversion  ConversionOutput=Bus copy
  OutBus : Outport  OutDataType=fixdt(1, 16)  OutScaling=2^0  InitialOutput=[0]
  wires:
  Bus Assignment1/1 -> OutBus/1
  Bus Selector/1 -> OperState: Driving/1(GBKind)  "<GBKind>"
  InBus/1 -> Bus Selector/1, Signal Conversion/1
  OperationFinished/1 -> Bus Assignment1/10
  Phase/1 -> Bus Assignment1/9
  OperState: Driving/1(BusOut) -> Bus Selector1/1  "VC_Bus"
  Signal Conversion/1 -> Bus Assignment1/1
  Bus Selector1/1 -> Bus Assignment1/2  "<Key>"
  Bus Selector1/2 -> Bus Assignment1/3  "<GearNo>"
  Bus Selector1/3 -> Bus Assignment1/4  "<SelectorCtrl>"
  Bus Selector1/4 -> Bus Assignment1/5  "<Gas>"
  Bus Selector1/5 -> Bus Assignment1/6  "<Clutch>"
  Bus Selector1/6 -> Bus Assignment1/7  "<Brake>"
  Bus Selector1/7 -> Bus Assignment1/8  "<BrakePark>"

== system MyVhclOperator_RTW/MyVhclOperator/Trg: OperState_Driving/OperState_PowerAccessory ==
  InBus : Inport  OutDataType=fixdt(1, 16)  OutScaling=2^0
  Action Port : ActionPort  ActionType=case
  Bus Assignment1 : BusAssignment  AssignedSignals=VCBus.Key,VCBus.GearNo,VCBus.SelectorCtrl,VCBus.Gas,VCBus.Clutch,VCBus.Brake,VCBus.BrakePark,Phase
  Bus Selector : BusSelector  OutputSignals=GBKind,Phase
  Bus Selector1 : BusSelector  OutputSignals=Key,GearNo,SelectorCtrl,Gas,Clutch,Brake,BrakePark
  OperState: PowerOn : Subsystem
  SetOutputAndWait : Subsystem
  Signal Conversion : SignalConversion  ConversionOutput=Bus copy
  OutBus : Outport  OutDataType=fixdt(1, 16)  OutScaling=2^0  InitialOutput=[0]
  wires:
  OperState: PowerOn/1(BusOut) -> Bus Selector1/1  "VC_Bus"
  SetOutputAndWait/1(PhaseOut) -> Bus Assignment1/9
  InBus/1 -> Bus Selector/1, Signal Conversion/1
  Bus Selector/1 -> OperState: PowerOn/1(GBKind)  "<GBKind>"
  Bus Assignment1/1 -> OutBus/1
  Bus Selector/2 -> SetOutputAndWait/1(PhaseIn)  "<Phase>"
  Signal Conversion/1 -> Bus Assignment1/1
  Bus Selector1/1 -> Bus Assignment1/2  "<Key>"
  Bus Selector1/2 -> Bus Assignment1/3  "<GearNo>"
  Bus Selector1/3 -> Bus Assignment1/4  "<SelectorCtrl>"
  Bus Selector1/4 -> Bus Assignment1/5  "<Gas>"
  Bus Selector1/5 -> Bus Assignment1/6  "<Clutch>"
  Bus Selector1/6 -> Bus Assignment1/7  "<Brake>"
  Bus Selector1/7 -> Bus Assignment1/8  "<BrakePark>"

== system MyVhclOperator_RTW/MyVhclOperator/Trg: OperState_Driving/OperState_PowerOff ==
  InBus : Inport  OutDataType=fixdt(1, 16)  OutScaling=2^0
  Action Port : ActionPort  ActionType=case
  Bus Assignment1 : BusAssignment  AssignedSignals=VCBus.Key,VCBus.GearNo,VCBus.SelectorCtrl,VCBus.Gas,VCBus.Clutch,VCBus.Brake,VCBus.BrakePark,Phase
  Bus Selector : BusSelector  OutputSignals=GBKind,Phase
  Bus Selector1 : BusSelector  OutputSignals=Key,GearNo,SelectorCtrl,Gas,Clutch,Brake,BrakePark
  OperState: PowerAcc : Subsystem
  SetOutputAndWait : Subsystem
  Signal Conversion : SignalConversion  ConversionOutput=Bus copy
  OutBus : Outport  OutDataType=fixdt(1, 16)  OutScaling=2^0  InitialOutput=[0]
  wires:
  Bus Selector/2 -> SetOutputAndWait/1(PhaseIn)  "<Phase>"
  Bus Assignment1/1 -> OutBus/1
  Bus Selector/1 -> OperState: PowerAcc/1(GBKind)  "<GBKind>"
  InBus/1 -> Bus Selector/1, Signal Conversion/1
  SetOutputAndWait/1(PhaseOut) -> Bus Assignment1/9
  OperState: PowerAcc/1(BusOut) -> Bus Selector1/1  "VC_Bus"
  Signal Conversion/1 -> Bus Assignment1/1
  Bus Selector1/1 -> Bus Assignment1/2  "<Key>"
  Bus Selector1/2 -> Bus Assignment1/3  "<GearNo>"
  Bus Selector1/3 -> Bus Assignment1/4  "<SelectorCtrl>"
  Bus Selector1/4 -> Bus Assignment1/5  "<Gas>"
  Bus Selector1/5 -> Bus Assignment1/6  "<Clutch>"
  Bus Selector1/6 -> Bus Assignment1/7  "<Brake>"
  Bus Selector1/7 -> Bus Assignment1/8  "<BrakePark>"

== system MyVhclOperator_RTW/MyVhclOperator/Trg: OperState_Driving/OperState_PowerOn ==
  InBus : Inport  OutDataType=fixdt(1, 16)  OutScaling=2^0
  Action Port : ActionPort  ActionType=case
  Bus Assignment1 : BusAssignment  AssignedSignals=VCBus.Key,VCBus.GearNo,VCBus.SelectorCtrl,VCBus.Gas,VCBus.Clutch,VCBus.Brake,VCBus.BrakePark,Phase
  Bus Selector : BusSelector  OutputSignals=GBKind,Phase
  Bus Selector1 : BusSelector  OutputSignals=Key,GearNo,SelectorCtrl,Gas,Clutch,Brake,BrakePark
  OperState: Starting : Subsystem
  SetOutputAndWait : Subsystem
  Signal Conversion : SignalConversion  ConversionOutput=Bus copy
  OutBus : Outport  OutDataType=fixdt(1, 16)  OutScaling=2^0  InitialOutput=[0]
  wires:
  InBus/1 -> Bus Selector/1, Signal Conversion/1
  Bus Selector/1 -> OperState: Starting/1(GBKind)  "<GBKind>"
  Bus Assignment1/1 -> OutBus/1
  Bus Selector/2 -> SetOutputAndWait/1(PhaseIn)  "<Phase>"
  SetOutputAndWait/1(PhaseOut) -> Bus Assignment1/9
  OperState: Starting/1(BusOut) -> Bus Selector1/1  "VC_Bus"
  Signal Conversion/1 -> Bus Assignment1/1
  Bus Selector1/1 -> Bus Assignment1/2  "<Key>"
  Bus Selector1/2 -> Bus Assignment1/3  "<GearNo>"
  Bus Selector1/3 -> Bus Assignment1/4  "<SelectorCtrl>"
  Bus Selector1/4 -> Bus Assignment1/5  "<Gas>"
  Bus Selector1/5 -> Bus Assignment1/6  "<Clutch>"
  Bus Selector1/6 -> Bus Assignment1/7  "<Brake>"
  Bus Selector1/7 -> Bus Assignment1/8  "<BrakePark>"

== system MyVhclOperator_RTW/MyVhclOperator/Trg: OperState_PowerOff/OperState_Absent ==
  InBus : Inport  OutDataType=fixdt(1, 16)  OutScaling=2^0
  Action Port : ActionPort  ActionType=case
  Bus Assignment : BusAssignment  AssignedSignals=VCBus.Key,VCBus.GearNo,VCBus.SelectorCtrl,VCBus.Gas,VCBus.Clutch,VCBus.Brake,VCBus.BrakePark
  Bus Selector : BusSelector  OutputSignals=GBKind
  Bus Selector1 : BusSelector  OutputSignals=Key,GearNo,SelectorCtrl,Gas,Clutch,Brake,BrakePark
  OperState: PowerOff : Subsystem
  Signal Conversion : SignalConversion  ConversionOutput=Bus copy
  OutBus : Outport  OutDataType=fixdt(1, 16)  OutScaling=2^0  InitialOutput=[0]
  wires:
  InBus/1 -> Bus Selector/1, Signal Conversion/1
  Bus Selector/1 -> OperState: PowerOff/1(GBKind)  "<GBKind>"
  Bus Assignment/1 -> OutBus/1
  OperState: PowerOff/1(BusOut) -> Bus Selector1/1  "VC_Bus"
  Signal Conversion/1 -> Bus Assignment/1
  Bus Selector1/1 -> Bus Assignment/2  "<Key>"
  Bus Selector1/2 -> Bus Assignment/3  "<GearNo>"
  Bus Selector1/3 -> Bus Assignment/4  "<SelectorCtrl>"
  Bus Selector1/4 -> Bus Assignment/5  "<Gas>"
  Bus Selector1/5 -> Bus Assignment/6  "<Clutch>"
  Bus Selector1/6 -> Bus Assignment/7  "<Brake>"
  Bus Selector1/7 -> Bus Assignment/8  "<BrakePark>"

== system MyVhclOperator_RTW/MyVhclOperator/Trg: OperState_PowerOff/OperState_Driving ==
  InBus : Inport  OutDataType=fixdt(1, 16)  OutScaling=2^0
  Action Port : ActionPort  ActionType=case
  Drive2Off : Subsystem
  OutBus : Outport  OutDataType=fixdt(1, 16)  OutScaling=2^0
  wires:
  Drive2Off/1(BusOut) -> OutBus/1
  InBus/1 -> Drive2Off/1(BusIn)

== system MyVhclOperator_RTW/MyVhclOperator/Trg: OperState_PowerOff/OperState_PowerAccessory ==
  InBus : Inport  OutDataType=fixdt(1, 16)  OutScaling=2^0
  Action Port : ActionPort  ActionType=case
  Bus Assignment1 : BusAssignment  AssignedSignals=VCBus.Key,VCBus.GearNo,VCBus.SelectorCtrl,VCBus.Gas,VCBus.Clutch,VCBus.Brake,VCBus.BrakePark,Phase
  Bus Selector : BusSelector  OutputSignals=GBKind,Phase
  Bus Selector1 : BusSelector  OutputSignals=Key,GearNo,SelectorCtrl,Gas,Clutch,Brake,BrakePark
  OperState: PowerOn : Subsystem
  SetOutputAndWait : Subsystem
  Signal Conversion : SignalConversion  ConversionOutput=Bus copy
  OutBus : Outport  OutDataType=fixdt(1, 16)  OutScaling=2^0  InitialOutput=[0]
  wires:
  SetOutputAndWait/1(PhaseOut) -> Bus Assignment1/9
  OperState: PowerOn/1(BusOut) -> Bus Selector1/1  "VC_Bus"
  Bus Selector/2 -> SetOutputAndWait/1(PhaseIn)  "<Phase>"
  Bus Assignment1/1 -> OutBus/1
  Bus Selector/1 -> OperState: PowerOn/1(GBKind)  "<GBKind>"
  InBus/1 -> Bus Selector/1, Signal Conversion/1
  Signal Conversion/1 -> Bus Assignment1/1
  Bus Selector1/1 -> Bus Assignment1/2  "<Key>"
  Bus Selector1/2 -> Bus Assignment1/3  "<GearNo>"
  Bus Selector1/3 -> Bus Assignment1/4  "<SelectorCtrl>"
  Bus Selector1/4 -> Bus Assignment1/5  "<Gas>"
  Bus Selector1/5 -> Bus Assignment1/6  "<Clutch>"
  Bus Selector1/6 -> Bus Assignment1/7  "<Brake>"
  Bus Selector1/7 -> Bus Assignment1/8  "<BrakePark>"

== system MyVhclOperator_RTW/MyVhclOperator/Trg: OperState_PowerOff/OperState_PowerOff ==
  InBus : Inport  OutDataType=fixdt(1, 16)  OutScaling=2^0
  Action Port : ActionPort  ActionType=case
  Bus Assignment1 : BusAssignment  AssignedSignals=VCBus.Key,VCBus.GearNo,VCBus.SelectorCtrl,VCBus.Gas,VCBus.Clutch,VCBus.Brake,VCBus.BrakePark,Phase,OperationFinished
  Bus Selector : BusSelector  OutputSignals=GBKind
  Bus Selector1 : BusSelector  OutputSignals=Key,GearNo,SelectorCtrl,Gas,Clutch,Brake,BrakePark
  OperState: PowerOff : Subsystem
  OperationFinished : Constant  OutDataType=fixdt(1, 16)  OutScaling=2^0
  Phase : Constant  Value=0  OutDataType=fixdt(1, 16)  OutScaling=2^0
  Signal Conversion : SignalConversion  ConversionOutput=Bus copy
  OutBus : Outport  OutDataType=fixdt(1, 16)  OutScaling=2^0  InitialOutput=[0]
  wires:
  InBus/1 -> Bus Selector/1, Signal Conversion/1
  Bus Selector/1 -> OperState: PowerOff/1(GBKind)  "<GBKind>"
  OperationFinished/1 -> Bus Assignment1/10
  Phase/1 -> Bus Assignment1/9
  OperState: PowerOff/1(BusOut) -> Bus Selector1/1  "VC_Bus"
  Bus Assignment1/1 -> OutBus/1
  Signal Conversion/1 -> Bus Assignment1/1
  Bus Selector1/1 -> Bus Assignment1/2  "<Key>"
  Bus Selector1/2 -> Bus Assignment1/3  "<GearNo>"
  Bus Selector1/3 -> Bus Assignment1/4  "<SelectorCtrl>"
  Bus Selector1/4 -> Bus Assignment1/5  "<Gas>"
  Bus Selector1/5 -> Bus Assignment1/6  "<Clutch>"
  Bus Selector1/6 -> Bus Assignment1/7  "<Brake>"
  Bus Selector1/7 -> Bus Assignment1/8  "<BrakePark>"

== system MyVhclOperator_RTW/MyVhclOperator/Trg: OperState_PowerOff/OperState_PowerOn ==
  InBus : Inport  OutDataType=fixdt(1, 16)  OutScaling=2^0
  Action Port : ActionPort  ActionType=case
  Bus Assignment1 : BusAssignment  AssignedSignals=VCBus.Key,VCBus.GearNo,VCBus.SelectorCtrl,VCBus.Gas,VCBus.Clutch,VCBus.Brake,VCBus.BrakePark,Phase
  Bus Selector : BusSelector  OutputSignals=GBKind,Phase
  Bus Selector1 : BusSelector  OutputSignals=Key,GearNo,SelectorCtrl,Gas,Clutch,Brake,BrakePark
  OperState: PowerOff : Subsystem
  SetOutputAndWait : Subsystem
  Signal Conversion : SignalConversion  ConversionOutput=Bus copy
  OutBus : Outport  OutDataType=fixdt(1, 16)  OutScaling=2^0  InitialOutput=[0]
  wires:
  Bus Assignment1/1 -> OutBus/1
  SetOutputAndWait/1(PhaseOut) -> Bus Assignment1/9
  OperState: PowerOff/1(BusOut) -> Bus Selector1/1  "VC_Bus"
  InBus/1 -> Bus Selector/1, Signal Conversion/1
  Bus Selector/1 -> OperState: PowerOff/1(GBKind)  "<GBKind>"
  Bus Selector/2 -> SetOutputAndWait/1(PhaseIn)  "<Phase>"
  Signal Conversion/1 -> Bus Assignment1/1
  Bus Selector1/1 -> Bus Assignment1/2  "<Key>"
  Bus Selector1/2 -> Bus Assignment1/3  "<GearNo>"
  Bus Selector1/3 -> Bus Assignment1/4  "<SelectorCtrl>"
  Bus Selector1/4 -> Bus Assignment1/5  "<Gas>"
  Bus Selector1/5 -> Bus Assignment1/6  "<Clutch>"
  Bus Selector1/6 -> Bus Assignment1/7  "<Brake>"
  Bus Selector1/7 -> Bus Assignment1/8  "<BrakePark>"

== system MyVhclOperator_RTW/MyVhclOperator/Trg: OperState_PowerOn/OperState_Absent ==
  InBus : Inport  OutDataType=fixdt(1, 16)  OutScaling=2^0
  Action Port : ActionPort  ActionType=case
  Bus Assignment : BusAssignment  AssignedSignals=VCBus.Key,VCBus.GearNo,VCBus.SelectorCtrl,VCBus.Gas,VCBus.Clutch,VCBus.Brake,VCBus.BrakePark
  Bus Selector : BusSelector  OutputSignals=GBKind
  Bus Selector1 : BusSelector  OutputSignals=Key,GearNo,SelectorCtrl,Gas,Clutch,Brake,BrakePark
  OperState: PowerOff : Subsystem
  Signal Conversion : SignalConversion  ConversionOutput=Bus copy
  OutBus : Outport  OutDataType=fixdt(1, 16)  OutScaling=2^0  InitialOutput=[0]
  wires:
  OperState: PowerOff/1(BusOut) -> Bus Selector1/1  "VC_Bus"
  Bus Assignment/1 -> OutBus/1
  Bus Selector/1 -> OperState: PowerOff/1(GBKind)  "<GBKind>"
  InBus/1 -> Bus Selector/1, Signal Conversion/1
  Signal Conversion/1 -> Bus Assignment/1
  Bus Selector1/1 -> Bus Assignment/2  "<Key>"
  Bus Selector1/2 -> Bus Assignment/3  "<GearNo>"
  Bus Selector1/3 -> Bus Assignment/4  "<SelectorCtrl>"
  Bus Selector1/4 -> Bus Assignment/5  "<Gas>"
  Bus Selector1/5 -> Bus Assignment/6  "<Clutch>"
  Bus Selector1/6 -> Bus Assignment/7  "<Brake>"
  Bus Selector1/7 -> Bus Assignment/8  "<BrakePark>"

== system MyVhclOperator_RTW/MyVhclOperator/Trg: OperState_PowerOn/OperState_Driving ==
  InBus : Inport  OutDataType=fixdt(1, 16)  OutScaling=2^0
  Action Port : ActionPort  ActionType=case
  Drive2Off : Subsystem
  OutBus : Outport  OutDataType=fixdt(1, 16)  OutScaling=2^0
  wires:
  Drive2Off/1(BusOut) -> OutBus/1
  InBus/1 -> Drive2Off/1(BusIn)

== system MyVhclOperator_RTW/MyVhclOperator/Trg: OperState_PowerOn/OperState_PowerAccessory ==
  InBus : Inport  OutDataType=fixdt(1, 16)  OutScaling=2^0
  Action Port : ActionPort  ActionType=case
  Bus Assignment1 : BusAssignment  AssignedSignals=VCBus.Key,VCBus.GearNo,VCBus.SelectorCtrl,VCBus.Gas,VCBus.Clutch,VCBus.Brake,VCBus.BrakePark,Phase
  Bus Selector : BusSelector  OutputSignals=GBKind,Phase
  Bus Selector1 : BusSelector  OutputSignals=Key,GearNo,SelectorCtrl,Gas,Clutch,Brake,BrakePark
  OperState: PowerOn : Subsystem
  SetOutputAndWait : Subsystem
  Signal Conversion : SignalConversion  ConversionOutput=Bus copy
  OutBus : Outport  OutDataType=fixdt(1, 16)  OutScaling=2^0  InitialOutput=[0]
  wires:
  Bus Selector/2 -> SetOutputAndWait/1(PhaseIn)  "<Phase>"
  Bus Assignment1/1 -> OutBus/1
  Bus Selector/1 -> OperState: PowerOn/1(GBKind)  "<GBKind>"
  InBus/1 -> Bus Selector/1, Signal Conversion/1
  SetOutputAndWait/1(PhaseOut) -> Bus Assignment1/9
  OperState: PowerOn/1(BusOut) -> Bus Selector1/1  "VC_Bus"
  Signal Conversion/1 -> Bus Assignment1/1
  Bus Selector1/1 -> Bus Assignment1/2  "<Key>"
  Bus Selector1/2 -> Bus Assignment1/3  "<GearNo>"
  Bus Selector1/3 -> Bus Assignment1/4  "<SelectorCtrl>"
  Bus Selector1/4 -> Bus Assignment1/5  "<Gas>"
  Bus Selector1/5 -> Bus Assignment1/6  "<Clutch>"
  Bus Selector1/6 -> Bus Assignment1/7  "<Brake>"
  Bus Selector1/7 -> Bus Assignment1/8  "<BrakePark>"

== system MyVhclOperator_RTW/MyVhclOperator/Trg: OperState_PowerOn/OperState_PowerOff ==
  InBus : Inport  OutDataType=fixdt(1, 16)  OutScaling=2^0
  Action Port : ActionPort  ActionType=case
  Bus Assignment1 : BusAssignment  AssignedSignals=VCBus.Key,VCBus.GearNo,VCBus.SelectorCtrl,VCBus.Gas,VCBus.Clutch,VCBus.Brake,VCBus.BrakePark,Phase
  Bus Selector : BusSelector  OutputSignals=GBKind,Phase
  Bus Selector1 : BusSelector  OutputSignals=Key,GearNo,SelectorCtrl,Gas,Clutch,Brake,BrakePark
  OperState: PowerAcc : Subsystem
  SetOutputAndWait : Subsystem
  Signal Conversion : SignalConversion  ConversionOutput=Bus copy
  OutBus : Outport  OutDataType=fixdt(1, 16)  OutScaling=2^0  InitialOutput=[0]
  wires:
  OperState: PowerAcc/1(BusOut) -> Bus Selector1/1  "VC_Bus"
  SetOutputAndWait/1(PhaseOut) -> Bus Assignment1/9
  InBus/1 -> Bus Selector/1, Signal Conversion/1
  Bus Selector/1 -> OperState: PowerAcc/1(GBKind)  "<GBKind>"
  Bus Assignment1/1 -> OutBus/1
  Bus Selector/2 -> SetOutputAndWait/1(PhaseIn)  "<Phase>"
  Signal Conversion/1 -> Bus Assignment1/1
  Bus Selector1/1 -> Bus Assignment1/2  "<Key>"
  Bus Selector1/2 -> Bus Assignment1/3  "<GearNo>"
  Bus Selector1/3 -> Bus Assignment1/4  "<SelectorCtrl>"
  Bus Selector1/4 -> Bus Assignment1/5  "<Gas>"
  Bus Selector1/5 -> Bus Assignment1/6  "<Clutch>"
  Bus Selector1/6 -> Bus Assignment1/7  "<Brake>"
  Bus Selector1/7 -> Bus Assignment1/8  "<BrakePark>"

== system MyVhclOperator_RTW/MyVhclOperator/Trg: OperState_PowerOn/OperState_PowerOn ==
  InBus : Inport  OutDataType=fixdt(1, 16)  OutScaling=2^0
  Action Port : ActionPort  ActionType=case
  Bus Assignment1 : BusAssignment  AssignedSignals=VCBus.Key,VCBus.GearNo,VCBus.SelectorCtrl,VCBus.Gas,VCBus.Clutch,VCBus.Brake,VCBus.BrakePark,Phase,OperationFinished
  Bus Selector : BusSelector  OutputSignals=GBKind
  Bus Selector1 : BusSelector  OutputSignals=Key,GearNo,SelectorCtrl,Gas,Clutch,Brake,BrakePark
  OperState: PowerOn : Subsystem
  OperationFinished : Constant  OutDataType=fixdt(1, 16)  OutScaling=2^0
  Phase : Constant  Value=0  OutDataType=fixdt(1, 16)  OutScaling=2^0
  Signal Conversion : SignalConversion  ConversionOutput=Bus copy
  OutBus : Outport  OutDataType=fixdt(1, 16)  OutScaling=2^0  InitialOutput=[0]
  wires:
  Bus Assignment1/1 -> OutBus/1
  Bus Selector/1 -> OperState: PowerOn/1(GBKind)  "<GBKind>"
  InBus/1 -> Bus Selector/1, Signal Conversion/1
  OperationFinished/1 -> Bus Assignment1/10
  Phase/1 -> Bus Assignment1/9
  OperState: PowerOn/1(BusOut) -> Bus Selector1/1  "VC_Bus"
  Signal Conversion/1 -> Bus Assignment1/1
  Bus Selector1/1 -> Bus Assignment1/2  "<Key>"
  Bus Selector1/2 -> Bus Assignment1/3  "<GearNo>"
  Bus Selector1/3 -> Bus Assignment1/4  "<SelectorCtrl>"
  Bus Selector1/4 -> Bus Assignment1/5  "<Gas>"
  Bus Selector1/5 -> Bus Assignment1/6  "<Clutch>"
  Bus Selector1/6 -> Bus Assignment1/7  "<Brake>"
  Bus Selector1/7 -> Bus Assignment1/8  "<BrakePark>"
